simulink model "MPPT_beta"  (Simulink 8.5)
settings: Solver=ode3  StartTime=0.0  StopTime=6  FixedStep=1e-3  RelTol=1e-3
InitFcn:
  | % Ponto de linearização
  | D = 0.5;
  | L = 0.1;
  | C = 0.01;
  | R = 10;
  | Vo = 24;
  | Leq = L/(1-D)^2;
  | N = 1/(1-D);
libraries: AvgModels x5, simulink x3
settings Model: Creator=Luigi2  LastModifiedBy=lgalo
settings OptimizationCC: InitFltsAndDblsToZero=on
settings DebuggingCC: SaveWithParameterizedLinksMsg=none  SolverPrmCheckMsg=warning  FcnCallInpInsideContextMsg=UseLocalSettings
settings GRTTargetCC: TargetFcnLib=ansi_tfl_tmw.mat
settings ConfigurationSet: Description=SimMechanics 2G

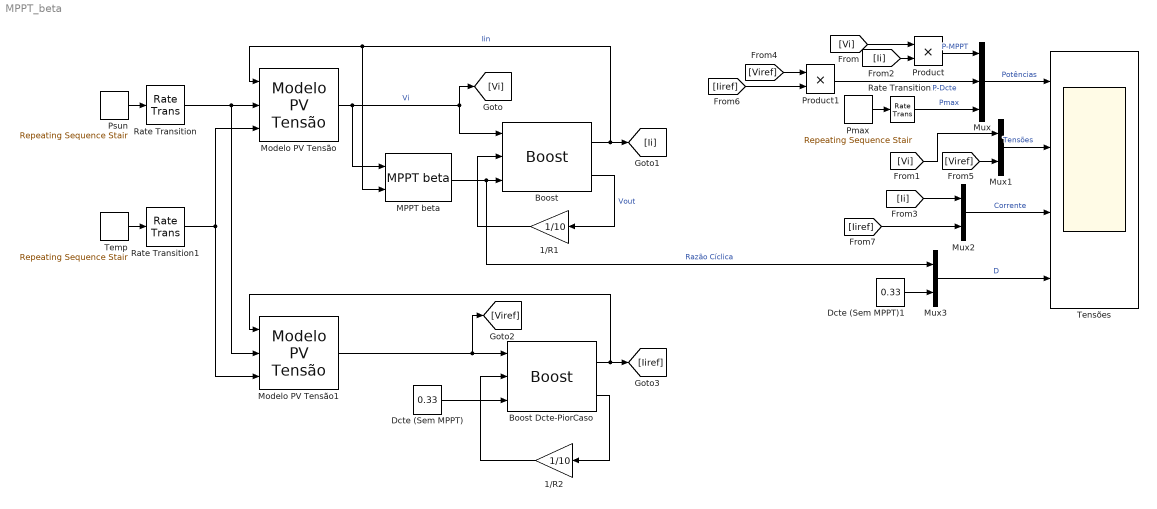
== system MPPT_beta ==
  1/R1 : Gain  Gain=1/10
  1/R2 : Gain  Gain=1/10
  Boost : AvgModels/Conversores Eletrônicos de Potência/Boost  L=0.1  RL=0  C=0.01  Edit_carga=24  Vini=0  Iini=0  Fs=20000  Vdon=0.7  Rdon=0  Vson=0  Rdson=0
  Boost Dcte-PiorCaso : AvgModels/Conversores Eletrônicos de Potência/Boost  L=0.1  RL=0  C=0.01  Edit_carga=24  Vini=0  Iini=0  Fs=20000  Vdon=0.7  Rdon=0  Vson=0  Rdson=0
  Dcte (Sem MPPT) : Constant  Value=0.33
  Dcte (Sem MPPT)1 : Constant  Value=0.33
  MPPT beta : AvgModels/MPPT/MPPT beta  betaref=-18  limsup=0.95  liminf=0  Kp=0.05  Ki=0.8
  Modelo PV Tensão : AvgModels/Modelo PV Tensão  Ms=1  Mp=1  Ns=54  Voc=0.6093  Isc=8.21  Tr=273 + 25  Rs=0.005  Rp=7  a=3.18e-3  n=1.2  k=1.38e-23  q=1.60e-19  EG=1.1
  Modelo PV Tensão1 : AvgModels/Modelo PV Tensão  Ms=1  Mp=1  Ns=54  Voc=0.6093  Isc=8.21  Tr=273 + 25  Rs=0.005  Rp=7  a=3.18e-3  n=1.2  k=1.38e-23  q=1.60e-19  EG=1.1
  Mux : Mux  Inputs=3
  Mux1 : Mux  Inputs=2
  Mux2 : Mux  Inputs=2
  Mux3 : Mux  Inputs=2
  Pmax : simulink/Sources/Repeating Sequence Stair  OutValues="[98.6721 187.4175  98.6721].'"  tsamp=2  OutMin=[]  OutMax=[]  OutDataTypeStr=double  OutputDataTypeScalingMode=double  OutDataType=fixdt(0,8)  ConRadixGroup=Best Precision: Vector-wise  OutScaling=2^-12
  Product : Product  RndMeth=Zero
  Product1 : Product  RndMeth=Zero
  Psun : simulink/Sources/Repeating Sequence Stair  OutValues=[500 1000 500].'  tsamp=2  OutMin=[]  OutMax=[]  OutDataTypeStr=double  OutputDataTypeScalingMode=double  OutDataType=fixdt(0,8)  ConRadixGroup=Best Precision: Vector-wise  OutScaling=2^-12
  Rate Transition : RateTransition
  Rate Transition1 : RateTransition
  Rate Transition2 : RateTransition
  Temp : simulink/Sources/Repeating Sequence Stair  OutValues=[25 40 25].'  tsamp=2  OutMin=[]  OutMax=[]  OutDataTypeStr=double  OutputDataTypeScalingMode=double  OutDataType=fixdt(0,8)  ConRadixGroup=Best Precision: Vector-wise  OutScaling=2^-12
  Tensões : Scope  NumInputPorts=4
      settings: TimeRange=6  YMin=-50~0~-2~0  YMax=200~40~8~0.5
  wires:
  Modelo PV Tensão/1 -> MPPT beta/1, [Vi], Boost/1  "Vi"
  Boost/2 -> 1/R1/1  "Vout"
  1/R1/1 -> Boost/2
  Boost/1 -> MPPT beta/2, Modelo PV Tensão/1, [Ii]  "Iin"
  MPPT beta/1 -> Mux3/1, Boost/3  "Razão Cíclica"
  Product/1 -> Mux/1  "P-MPPT"
  Pmax/1 -> Rate Transition2/1
  Mux/1 -> Tensões/1  "Potências"
  Psun/1 -> Rate Transition/1
  Temp/1 -> Rate Transition1/1
  Rate Transition/1 -> Modelo PV Tensão1/2, Modelo PV Tensão/2
  Rate Transition1/1 -> Modelo PV Tensão/3, Modelo PV Tensão1/3
  Boost Dcte-PiorCaso/2 -> 1/R2/1
  1/R2/1 -> Boost Dcte-PiorCaso/2
  Boost Dcte-PiorCaso/1 -> [Iiref], Modelo PV Tensão1/1
  Product1/1 -> Mux/2  "P-Dcte"
  Dcte (Sem MPPT)/1 -> Boost Dcte-PiorCaso/3
  Modelo PV Tensão1/1 -> [Viref], Boost Dcte-PiorCaso/1
  Rate Transition2/1 -> Mux/3  "Pmax"
  Mux1/1 -> Tensões/2  "Tensões"
  Mux2/1 -> Tensões/3  "Corrente"
  [Vi] -> Product/1
  [Vi] -> Mux1/1
  [Ii] -> Product/2
  [Ii] -> Mux2/1
  Dcte (Sem MPPT)1/1 -> Mux3/2
  Mux3/1 -> Tensões/4  "D"
  [Viref] -> Product1/1
  [Viref] -> Mux1/2
  [Iiref] -> Product1/2
  [Iiref] -> Mux2/2
